simulink subsystem "Qmatrix"  (R2024b)
settings: Solver=VariableStepAuto  StartTime=0.0  StopTime=10.0  RelTol=1e-3
settings Model: Creator=ricca  LastModifiedBy=ricca

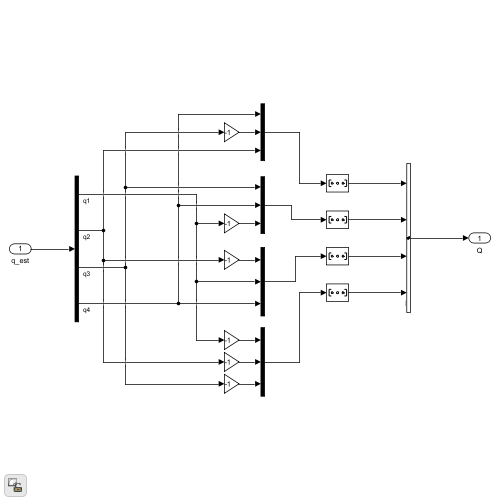
[thumbnail: Simulink's stored preview of the top-level diagram]
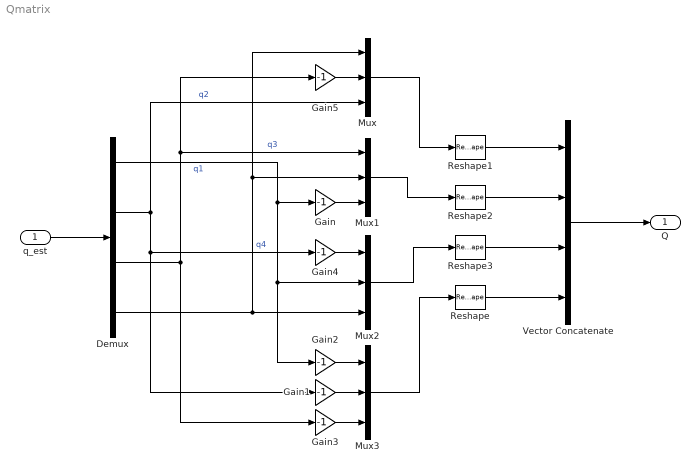
== system Qmatrix ==
  q_est : Inport
  Demux : Demux
  Gain{,1..5} (6 alike) : Gain  Gain=-1
  Mux{,1..3} (4 alike) : Mux  Inputs=3
  Reshape{,1..3} (4 alike) : Reshape  OutputDimensionality=Row vector (2-D)
  Vector Concatenate : Concatenate  NumInputs=4  Mode=Multidimensional array
  Q : Outport
  wires:
  Demux/1 -> Gain/1, Mux2/2, Gain2/1  "q1"
  Demux/2 -> Mux/3, Gain4/1, Gain1/1  "q2"
  Demux/3 -> Gain3/1, Gain5/1, Mux1/1  "q3"
  Demux/4 -> Mux2/3, Mux/1, Mux1/2  "q4"
  Vector Concatenate/1 -> Q/1
  Gain5/1 -> Mux/2
  Gain/1 -> Mux1/3
  Gain4/1 -> Mux2/1
  Gain3/1 -> Mux3/3
  Gain2/1 -> Mux3/1
  Gain1/1 -> Mux3/2
  Mux/1 -> Reshape1/1
  Mux1/1 -> Reshape2/1
  Mux2/1 -> Reshape3/1
  Mux3/1 -> Reshape/1
  Reshape/1 -> Vector Concatenate/4
  Reshape3/1 -> Vector Concatenate/3
  Reshape2/1 -> Vector Concatenate/2
  Reshape1/1 -> Vector Concatenate/1
  q_est/1 -> Demux/1
